simulink model "Exercitiul7"  (R2016a)
settings: Solver=VariableStepDiscrete  StartTime=0.0  StopTime=100  RelTol=1e-3
undefined symbols (not defined in the file): m, n
settings Model: Creator=Cristina  LastModifiedBy=Cristina

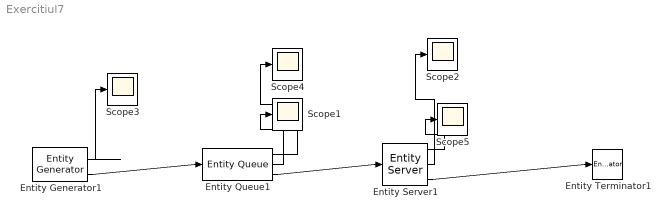
== system Exercitiul7 ==
  Entity Generator1 : EntityGenerator  OutputPortMessageModes=n,m  TimeSource=MATLAB action  IntergenerationTimeAction=dt = exprnd(0.2);  AttributeName=ServiceTime  NumberEntitiesDeparted=on  EntityType=Structured  EntityTypeName=Entity
      settings: OutputPortMap=o0,o3
  Entity Queue1 : EntityQueue  InputPortMessageModes=m  OutputPortMessageModes=n,n,m  NumberEntitiesDeparted=on  NumberEntitiesInBlock=on
      settings: OutputPortMap=o0,o1,o5
  Entity Server1 : EntityServer  InputPortMessageModes=m  OutputPortMessageModes=n,n,m  Capacity=inf  ServiceTimeSource=Attribute  ServiceTimeValue=1  ServiceTimeAction=dt = (1.2-0.8) * rand + 0.8  NumberEntitiesDeparted=on  NumberEntitiesInBlock=on
      settings: OutputPortMap=o0,o1,o9
  Entity Terminator1 : EntityTerminator  InputPortMessageModes=m
  Scope{1..5} (5 alike) : Scope
  wires:
  Entity Generator1/2 -> Entity Queue1/1
  Entity Queue1/3 -> Entity Server1/1
  Entity Server1/3 -> Entity Terminator1/1
  Entity Generator1/1 -> Scope3/1
  Entity Server1/1 -> Scope5/1
  Entity Queue1/2 -> Scope4/1
  Entity Queue1/1 -> Scope1/1
  Entity Server1/2 -> Scope2/1
